simulink model "simple_double_argon"  (Simulink 10.0)
settings: Solver=ode15s  StartTime=0.0  StopTime=3600*24  RelTol=1e-3  EnableMultiTasking=on
libraries: fl_lib x42, nesl_utility x9
settings Model: Creator=jlanfrey  LastModifiedBy=Ivan
settings DataIOCC: LimitDataPoints=on  SignalLoggingSaveFormat=ModelDataLogs
settings OptimizationCC: ExpressionDepthLimit=2147483647
settings DebuggingCC: SolverPrmCheckMsg=warning  FcnCallInpInsideContextMsg=warning  StateNameClashWarn=warning
settings GRTTargetCC: GeneratePreprocessorConditionals=Disable all
settings ConfigComp: CovExternalEMLEnable=off
settings SimscapeCC: SimscapeNormalizeSystem=off

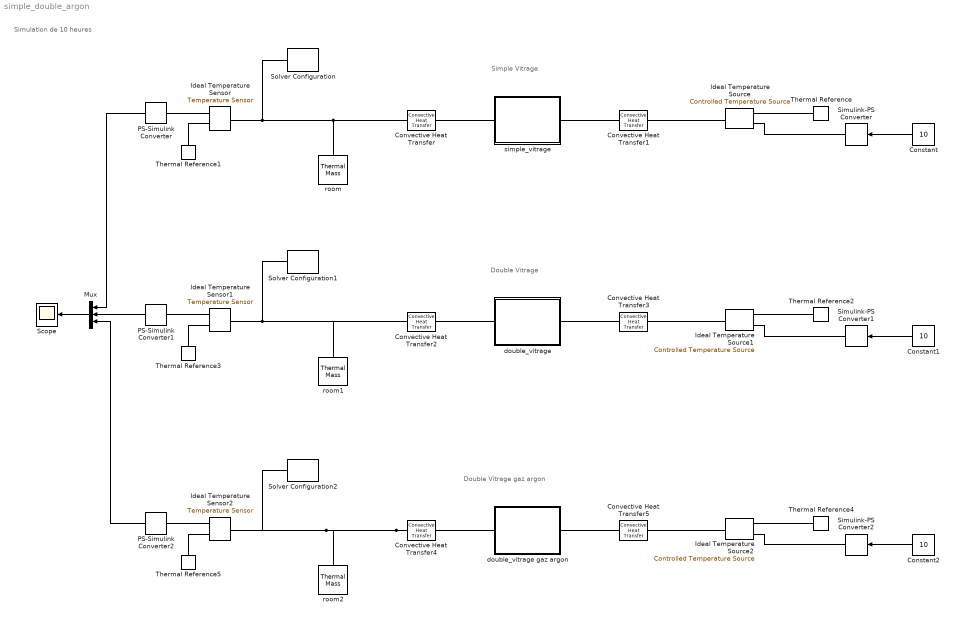
== system simple_double_argon ==
  note: Double Vitrage
  note: Simple Vitrage
  note: Simulation de 10 heures
  note: Double Vitrage gaz argon
  Constant : Constant  Value=10
  Constant1 : Constant  Value=10
  Constant2 : Constant  Value=10
  Convective Heat Transfer : fl_lib/Thermal/Thermal Elements/Convective Heat Transfer  area=0.6*1 m^2  heat_tr_coeff=1/0.13 W/(m^2 * K)  T_specify=off  T_priority=None  T=0 K  T_nominal_specify=off  T_nominal_unit=K  T_nominal_value=1  Q_specify=off  Q_priority=None  Q=0 J/s  Q_nominal_specify=off  Q_nominal_unit=J/s  Q_nominal_value=1
  Convective Heat Transfer1 : fl_lib/Thermal/Thermal Elements/Convective Heat Transfer  area=0.6*1 m^2  heat_tr_coeff=1/0.04 W/(m^2 * K)  T_specify=off  T_priority=None  T=0 K  T_nominal_specify=off  T_nominal_unit=K  T_nominal_value=1  Q_specify=off  Q_priority=None  Q=0 J/s  Q_nominal_specify=off  Q_nominal_unit=J/s  Q_nominal_value=1
  Convective Heat Transfer2 : fl_lib/Thermal/Thermal Elements/Convective Heat Transfer  area=0.6*1 m^2  heat_tr_coeff=1/0.13 W/(m^2 * K)  T_specify=off  T_priority=None  T=0 K  T_nominal_specify=off  T_nominal_unit=K  T_nominal_value=1  Q_specify=off  Q_priority=None  Q=0 J/s  Q_nominal_specify=off  Q_nominal_unit=J/s  Q_nominal_value=1
  Convective Heat Transfer3 : fl_lib/Thermal/Thermal Elements/Convective Heat Transfer  area=0.6*1 m^2  heat_tr_coeff=1/0.04 W/(m^2 * K)  T_specify=off  T_priority=None  T=0 K  T_nominal_specify=off  T_nominal_unit=K  T_nominal_value=1  Q_specify=off  Q_priority=None  Q=0 J/s  Q_nominal_specify=off  Q_nominal_unit=J/s  Q_nominal_value=1
  Convective Heat Transfer4 : fl_lib/Thermal/Thermal Elements/Convective Heat Transfer  area=0.6*1 m^2  heat_tr_coeff=1/0.13 W/(m^2 * K)  T_specify=off  T_priority=None  T=0 K  T_nominal_specify=off  T_nominal_unit=K  T_nominal_value=1  Q_specify=off  Q_priority=None  Q=0 J/s  Q_nominal_specify=off  Q_nominal_unit=J/s  Q_nominal_value=1
  Convective Heat Transfer5 : fl_lib/Thermal/Thermal Elements/Convective Heat Transfer  area=0.6*1 m^2  heat_tr_coeff=1/0.04 W/(m^2 * K)  T_specify=off  T_priority=None  T=0 K  T_nominal_specify=off  T_nominal_unit=K  T_nominal_value=1  Q_specify=off  Q_priority=None  Q=0 J/s  Q_nominal_specify=off  Q_nominal_unit=J/s  Q_nominal_value=1
  Ideal Temperature Sensor : fl_lib/Thermal/Thermal Sensors/Temperature Sensor
  Ideal Temperature Sensor1 : fl_lib/Thermal/Thermal Sensors/Temperature Sensor
  Ideal Temperature Sensor2 : fl_lib/Thermal/Thermal Sensors/Temperature Sensor
  Ideal Temperature Source : fl_lib/Thermal/Thermal Sources/Controlled Temperature Source
      settings: SourceProductName=Simscape
  Ideal Temperature Source1 : fl_lib/Thermal/Thermal Sources/Controlled Temperature Source
      settings: SourceProductName=Simscape
  Ideal Temperature Source2 : fl_lib/Thermal/Thermal Sources/Controlled Temperature Source
      settings: SourceProductName=Simscape
  Mux : Mux  Inputs=3
  PS-Simulink Converter : nesl_utility/PS-Simulink Converter  PhysicalDomain=network_engine_domain  SubClassName=ps_output  LeftPortType=input  RightPortType=output  PseudoPeriodic=off  Frequencies=[]  Unit=degC  AffineConversion=on
  PS-Simulink Converter1 : nesl_utility/PS-Simulink Converter  PhysicalDomain=network_engine_domain  SubClassName=ps_output  LeftPortType=input  RightPortType=output  PseudoPeriodic=off  Frequencies=[]  Unit=degC  AffineConversion=on
  PS-Simulink Converter2 : nesl_utility/PS-Simulink Converter  PhysicalDomain=network_engine_domain  SubClassName=ps_output  LeftPortType=input  RightPortType=output  PseudoPeriodic=off  Frequencies=[]  Unit=degC  AffineConversion=on
  Scope : Scope
  Simulink-PS Converter : nesl_utility/Simulink-PS Converter  PhysicalDomain=network_engine_domain  SubClassName=ps_input  LeftPortType=input  RightPortType=output  PseudoPeriodic=off  Frequencies=[]  NoiseDistribution=none  NoiseParameters=[]  Unit=degC  AffineConversion=on  FilteringAndDerivatives=zero  SimscapeFilterOrder=1  InputFilterTimeConstant=.001  UdotUserProvided=0
  Simulink-PS Converter1 : nesl_utility/Simulink-PS Converter  PhysicalDomain=network_engine_domain  SubClassName=ps_input  LeftPortType=input  RightPortType=output  PseudoPeriodic=off  Frequencies=[]  NoiseDistribution=none  NoiseParameters=[]  Unit=degC  AffineConversion=on  FilteringAndDerivatives=zero  SimscapeFilterOrder=1  InputFilterTimeConstant=.001  UdotUserProvided=0
  Simulink-PS Converter2 : nesl_utility/Simulink-PS Converter  PhysicalDomain=network_engine_domain  SubClassName=ps_input  LeftPortType=input  RightPortType=output  PseudoPeriodic=off  Frequencies=[]  NoiseDistribution=none  NoiseParameters=[]  Unit=degC  AffineConversion=on  FilteringAndDerivatives=zero  SimscapeFilterOrder=1  InputFilterTimeConstant=.001  UdotUserProvided=0
  Solver Configuration : nesl_utility/Solver Configuration  PhysicalDomain=network_engine_domain  SubClassName=solver  LeftPortType=input  RightPortType=generic  Tones=[]  Harmonics=[]  SimulateNoise=off  Profile=off  UseLocalSampling=off  EnableSwitchedLinearOptims=on  FrequencyDomain=off  UseCCode=off  RelTol=0.001  AbsTol=1e-06  MinStep=1e-09  ToWorkspace=off  RevertToSquareIcSolve=off  NumHomotopyIterations=100  PhasorMode=off  PhasorModeNumHarmonics=1  DoDC=off  ResidualTolerance=1e-9  UseLocalSolver=off  LocalSolverChoice=NE_BACKWARD_EULER_ADVANCER  LocalSolverSampleTime=.001  DoFixedCost=off  MaxNonlinIter=3  MaxModeIter=2  LinearAlgebra=Sparse  EquationFormulation=NE_TIME_EF  DelaysMemoryBudget=1024  AutomaticFiltering=on  FilteringTimeConstant=0.001  PartitionStorageMethod=AS_NEEDED  PartitionMemoryBudget=1024  PartitionMethod=FAST
  Solver Configuration1 : nesl_utility/Solver Configuration  PhysicalDomain=network_engine_domain  SubClassName=solver  LeftPortType=input  RightPortType=generic  Tones=[]  Harmonics=[]  SimulateNoise=off  Profile=off  UseLocalSampling=off  EnableSwitchedLinearOptims=on  FrequencyDomain=off  UseCCode=off  RelTol=0.001  AbsTol=1e-06  MinStep=1e-09  ToWorkspace=off  RevertToSquareIcSolve=off  NumHomotopyIterations=100  PhasorMode=off  PhasorModeNumHarmonics=1  DoDC=off  ResidualTolerance=1e-9  UseLocalSolver=off  LocalSolverChoice=NE_BACKWARD_EULER_ADVANCER  LocalSolverSampleTime=.001  DoFixedCost=off  MaxNonlinIter=3  MaxModeIter=2  LinearAlgebra=Sparse  EquationFormulation=NE_TIME_EF  DelaysMemoryBudget=1024  AutomaticFiltering=on  FilteringTimeConstant=0.001  PartitionStorageMethod=AS_NEEDED  PartitionMemoryBudget=1024  PartitionMethod=FAST
  Solver Configuration2 : nesl_utility/Solver Configuration  PhysicalDomain=network_engine_domain  SubClassName=solver  LeftPortType=input  RightPortType=generic  Tones=[]  Harmonics=[]  SimulateNoise=off  Profile=off  UseLocalSampling=off  EnableSwitchedLinearOptims=on  FrequencyDomain=off  UseCCode=off  RelTol=0.001  AbsTol=1e-06  MinStep=1e-09  ToWorkspace=off  RevertToSquareIcSolve=off  NumHomotopyIterations=100  PhasorMode=off  PhasorModeNumHarmonics=1  DoDC=off  ResidualTolerance=1e-9  UseLocalSolver=off  LocalSolverChoice=NE_BACKWARD_EULER_ADVANCER  LocalSolverSampleTime=.001  DoFixedCost=off  MaxNonlinIter=3  MaxModeIter=2  LinearAlgebra=Sparse  EquationFormulation=NE_TIME_EF  DelaysMemoryBudget=1024  AutomaticFiltering=on  FilteringTimeConstant=0.001  PartitionStorageMethod=AS_NEEDED  PartitionMemoryBudget=1024  PartitionMethod=FAST
  Thermal Reference{,1..5} (6 alike) : fl_lib/Thermal/Thermal Elements/Thermal Reference
  double_vitrage : Subsystem
  double_vitrage gaz argon : Subsystem
  room : fl_lib/Thermal/Thermal Elements/Thermal Mass  mass=1.204*10*2.5 kg  sp_heat=1004 J/kg/K  T_specify=on  T_priority=High  T=20 degC  T_nominal_specify=off  T_nominal_unit=K  T_nominal_value=1  Q_specify=off  Q_priority=None  Q=0 J/s  Q_nominal_specify=off  Q_nominal_unit=J/s  Q_nominal_value=1
  room1 : fl_lib/Thermal/Thermal Elements/Thermal Mass  mass=1.204*10*2.5 kg  sp_heat=1004 J/kg/K  T_specify=on  T_priority=High  T=20 degC  T_nominal_specify=off  T_nominal_unit=K  T_nominal_value=1  Q_specify=off  Q_priority=None  Q=0 J/s  Q_nominal_specify=off  Q_nominal_unit=J/s  Q_nominal_value=1
  room2 : fl_lib/Thermal/Thermal Elements/Thermal Mass  mass=1.204*10*2.5 kg  sp_heat=1004 J/kg/K  T_specify=on  T_priority=High  T=20 degC  T_nominal_specify=off  T_nominal_unit=K  T_nominal_value=1  Q_specify=off  Q_priority=None  Q=0 J/s  Q_nominal_specify=off  Q_nominal_unit=J/s  Q_nominal_value=1
  simple_vitrage : Subsystem
  wires:
  PS-Simulink Converter/1 -> Mux/1
  Constant/1 -> Simulink-PS Converter/1
  PS-Simulink Converter1/1 -> Mux/2
  Constant1/1 -> Simulink-PS Converter1/1
  Mux/1 -> Scope/1
  Constant2/1 -> Simulink-PS Converter2/1
  PS-Simulink Converter2/1 -> Mux/3
  connections:
  Thermal Reference2/LConn1 -- Ideal Temperature Source1/RConn2
  Simulink-PS Converter1/RConn1 -- Ideal Temperature Source1/RConn1
  Thermal Reference/LConn1 -- Ideal Temperature Source/RConn2
  Simulink-PS Converter/RConn1 -- Ideal Temperature Source/RConn1
  PS-Simulink Converter1/LConn1 -- Ideal Temperature Sensor1/RConn2
  Thermal Reference3/LConn1 -- Ideal Temperature Sensor1/RConn1
  PS-Simulink Converter/LConn1 -- Ideal Temperature Sensor/RConn2
  Thermal Reference1/LConn1 -- Ideal Temperature Sensor/RConn1
  Ideal Temperature Source1/LConn1 -- Convective Heat Transfer3/RConn1
  Convective Heat Transfer3/LConn1 -- double_vitrage/RConn1
  Convective Heat Transfer2/RConn1 -- double_vitrage/LConn1
  Solver Configuration1/RConn1 -- Ideal Temperature Sensor1/LConn1 -- room1/LConn1 -- Convective Heat Transfer2/LConn1
  Ideal Temperature Source/LConn1 -- Convective Heat Transfer1/RConn1
  Convective Heat Transfer1/LConn1 -- simple_vitrage/RConn1
  Convective Heat Transfer/RConn1 -- simple_vitrage/LConn1
  room/LConn1 -- Solver Configuration/RConn1 -- Ideal Temperature Sensor/LConn1 -- Convective Heat Transfer/LConn1
  Convective Heat Transfer4/LConn1 -- room2/LConn1 -- Solver Configuration2/RConn1 -- Ideal Temperature Sensor2/LConn1
  Thermal Reference5/LConn1 -- Ideal Temperature Sensor2/RConn1
  PS-Simulink Converter2/LConn1 -- Ideal Temperature Sensor2/RConn2
  Thermal Reference4/LConn1 -- Ideal Temperature Source2/RConn2
  Simulink-PS Converter2/RConn1 -- Ideal Temperature Source2/RConn1
  Ideal Temperature Source2/LConn1 -- Convective Heat Transfer5/RConn1
  Convective Heat Transfer5/LConn1 -- double_vitrage gaz argon/RConn1
  Convective Heat Transfer4/RConn1 -- double_vitrage gaz argon/LConn1

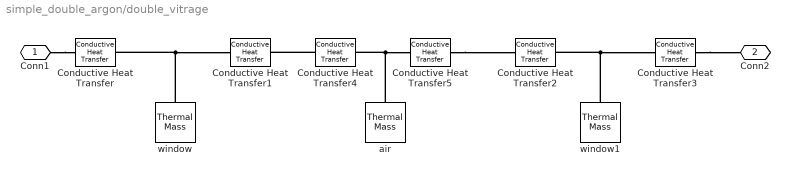
== system simple_double_argon/double_vitrage ==
  Conductive Heat Transfer{,1..3} (4 alike) : fl_lib/Thermal/Thermal Elements/Conductive Heat Transfer  area=0.6*1 m^2  thickness=2 mm  th_cond=1.2 W/(m*K)  T_specify=off  T_priority=None  T=0 K  T_nominal_specify=off  T_nominal_unit=K  T_nominal_value=1  Q_specify=off  Q_priority=None  Q=0 J/s  Q_nominal_specify=off  Q_nominal_unit=J/s  Q_nominal_value=1
      settings: SourceProductName=Simscape
  Conductive Heat Transfer4 : fl_lib/Thermal/Thermal Elements/Conductive Heat Transfer  area=0.6*1 m^2  thickness=6 mm  th_cond=0.0262 W/(m*K)  T_specify=off  T_priority=None  T=0 K  T_nominal_specify=off  T_nominal_unit=K  T_nominal_value=1  Q_specify=off  Q_priority=None  Q=0 J/s  Q_nominal_specify=off  Q_nominal_unit=J/s  Q_nominal_value=1
      settings: SourceProductName=Simscape
  Conductive Heat Transfer5 : fl_lib/Thermal/Thermal Elements/Conductive Heat Transfer  area=0.6*1 m^2  thickness=6 mm  th_cond=0.0262 W/(m*K)  T_specify=off  T_priority=None  T=0 K  T_nominal_specify=off  T_nominal_unit=K  T_nominal_value=1  Q_specify=off  Q_priority=None  Q=0 J/s  Q_nominal_specify=off  Q_nominal_unit=J/s  Q_nominal_value=1
      settings: SourceProductName=Simscape
  air : fl_lib/Thermal/Thermal Elements/Thermal Mass  mass=0.6*1*1.204 kg  sp_heat=1004 J/kg/K  T_specify=on  T_priority=High  T=20 degC  T_nominal_specify=off  T_nominal_unit=K  T_nominal_value=1  Q_specify=off  Q_priority=None  Q=0 J/s  Q_nominal_specify=off  Q_nominal_unit=J/s  Q_nominal_value=1
  window : fl_lib/Thermal/Thermal Elements/Thermal Mass  mass=0.6*1*4e-3*2530 kg  sp_heat=720 J/kg/K  T_specify=on  T_priority=High  T=20 degC  T_nominal_specify=off  T_nominal_unit=K  T_nominal_value=1  Q_specify=off  Q_priority=None  Q=0 J/s  Q_nominal_specify=off  Q_nominal_unit=J/s  Q_nominal_value=1
  window1 : fl_lib/Thermal/Thermal Elements/Thermal Mass  mass=0.6*1*4e-3*2530 kg  sp_heat=720 J/kg/K  T_specify=on  T_priority=High  T=20 degC  T_nominal_specify=off  T_nominal_unit=K  T_nominal_value=1  Q_specify=off  Q_priority=None  Q=0 J/s  Q_nominal_specify=off  Q_nominal_unit=J/s  Q_nominal_value=1
  Conn1 : PMIOPort  Side=Left
  Conn2 : PMIOPort  Port=2  Side=Right
  connections:
  Conn1/RConn1 -- Conductive Heat Transfer/LConn1
  window/LConn1 -- Conductive Heat Transfer/RConn1 -- Conductive Heat Transfer1/LConn1
  window1/LConn1 -- Conductive Heat Transfer3/LConn1 -- Conductive Heat Transfer2/RConn1
  Conductive Heat Transfer3/RConn1 -- Conn2/RConn1
  Conductive Heat Transfer4/LConn1 -- Conductive Heat Transfer1/RConn1
  Conductive Heat Transfer5/RConn1 -- Conductive Heat Transfer2/LConn1
  air/LConn1 -- Conductive Heat Transfer4/RConn1 -- Conductive Heat Transfer5/LConn1

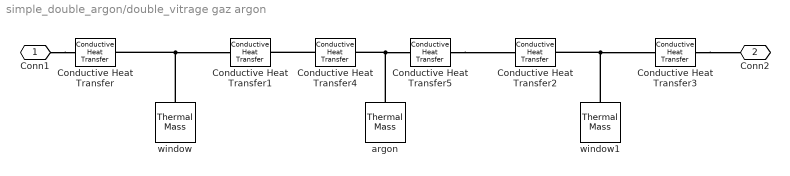
== system simple_double_argon/double_vitrage gaz argon ==
  Conductive Heat Transfer{,1..3} (4 alike) : fl_lib/Thermal/Thermal Elements/Conductive Heat Transfer  area=0.6*1 m^2  thickness=2 mm  th_cond=1.2 W/(m*K)  T_specify=off  T_priority=None  T=0 K  T_nominal_specify=off  T_nominal_unit=K  T_nominal_value=1  Q_specify=off  Q_priority=None  Q=0 J/s  Q_nominal_specify=off  Q_nominal_unit=J/s  Q_nominal_value=1
      settings: SourceProductName=Simscape
  Conductive Heat Transfer4 : fl_lib/Thermal/Thermal Elements/Conductive Heat Transfer  area=0.6*1 m^2  thickness=6 mm  th_cond="0.01772  W/(m*K)"  T_specify=off  T_priority=None  T=0 K  T_nominal_specify=off  T_nominal_unit=K  T_nominal_value=1  Q_specify=off  Q_priority=None  Q=0 J/s  Q_nominal_specify=off  Q_nominal_unit=J/s  Q_nominal_value=1
      settings: SourceProductName=Simscape
  Conductive Heat Transfer5 : fl_lib/Thermal/Thermal Elements/Conductive Heat Transfer  area=0.6*1 m^2  thickness=6 mm  th_cond="0.01772  W/(m*K)"  T_specify=off  T_priority=None  T=0 K  T_nominal_specify=off  T_nominal_unit=K  T_nominal_value=1  Q_specify=off  Q_priority=None  Q=0 J/s  Q_nominal_specify=off  Q_nominal_unit=J/s  Q_nominal_value=1
      settings: SourceProductName=Simscape
  argon : fl_lib/Thermal/Thermal Elements/Thermal Mass  mass=0.6*1*1.783 kg  sp_heat=320 J/kg/K  T_specify=on  T_priority=High  T=20 degC  T_nominal_specify=off  T_nominal_unit=K  T_nominal_value=1  Q_specify=off  Q_priority=None  Q=0 J/s  Q_nominal_specify=off  Q_nominal_unit=J/s  Q_nominal_value=1
  window : fl_lib/Thermal/Thermal Elements/Thermal Mass  mass=0.6*1*4e-3*2530 kg  sp_heat=720 J/kg/K  T_specify=on  T_priority=High  T=20 degC  T_nominal_specify=off  T_nominal_unit=K  T_nominal_value=1  Q_specify=off  Q_priority=None  Q=0 J/s  Q_nominal_specify=off  Q_nominal_unit=J/s  Q_nominal_value=1
  window1 : fl_lib/Thermal/Thermal Elements/Thermal Mass  mass=0.6*1*4e-3*2530 kg  sp_heat=720 J/kg/K  T_specify=on  T_priority=High  T=20 degC  T_nominal_specify=off  T_nominal_unit=K  T_nominal_value=1  Q_specify=off  Q_priority=None  Q=0 J/s  Q_nominal_specify=off  Q_nominal_unit=J/s  Q_nominal_value=1
  Conn1 : PMIOPort  Side=Left
  Conn2 : PMIOPort  Port=2  Side=Right
  connections:
  Conn1/RConn1 -- Conductive Heat Transfer/LConn1
  window/LConn1 -- Conductive Heat Transfer/RConn1 -- Conductive Heat Transfer1/LConn1
  window1/LConn1 -- Conductive Heat Transfer3/LConn1 -- Conductive Heat Transfer2/RConn1
  Conductive Heat Transfer3/RConn1 -- Conn2/RConn1
  Conductive Heat Transfer4/LConn1 -- Conductive Heat Transfer1/RConn1
  Conductive Heat Transfer5/RConn1 -- Conductive Heat Transfer2/LConn1
  argon/LConn1 -- Conductive Heat Transfer4/RConn1 -- Conductive Heat Transfer5/LConn1

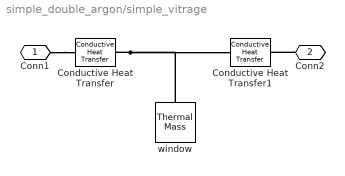
== system simple_double_argon/simple_vitrage ==
  Conductive Heat Transfer : fl_lib/Thermal/Thermal Elements/Conductive Heat Transfer  area=0.6*1 m^2  thickness=1.5 mm  th_cond=1.2 W/(m*K)  T_specify=off  T_priority=None  T=0 K  T_nominal_specify=off  T_nominal_unit=K  T_nominal_value=1  Q_specify=off  Q_priority=None  Q=0 J/s  Q_nominal_specify=off  Q_nominal_unit=J/s  Q_nominal_value=1
      settings: SourceProductName=Simscape
  Conductive Heat Transfer1 : fl_lib/Thermal/Thermal Elements/Conductive Heat Transfer  area=0.6*1 m^2  thickness=1.5 mm  th_cond=1.2 W/(m*K)  T_specify=off  T_priority=None  T=0 K  T_nominal_specify=off  T_nominal_unit=K  T_nominal_value=1  Q_specify=off  Q_priority=None  Q=0 J/s  Q_nominal_specify=off  Q_nominal_unit=J/s  Q_nominal_value=1
      settings: SourceProductName=Simscape
  window : fl_lib/Thermal/Thermal Elements/Thermal Mass  mass=0.6*1*3e-3*2530 kg  sp_heat=720 J/kg/K  T_specify=on  T_priority=High  T=20 degC  T_nominal_specify=off  T_nominal_unit=K  T_nominal_value=1  Q_specify=off  Q_priority=None  Q=0 J/s  Q_nominal_specify=off  Q_nominal_unit=J/s  Q_nominal_value=1
  Conn1 : PMIOPort  Side=Left
  Conn2 : PMIOPort  Port=2  Side=Right
  connections:
  Conductive Heat Transfer/RConn1 -- Conductive Heat Transfer1/LConn1 -- window/LConn1
  Conn1/RConn1 -- Conductive Heat Transfer/LConn1
  Conn2/RConn1 -- Conductive Heat Transfer1/RConn1
